simulink model "demo_zynq"  (R2019b)
settings: Solver=FixedStepAuto  StartTime=0.0  StopTime=0.02  RelTol=1e-3  EnableMultiTasking=on
InitFcn:
  | Ts_FPGA = 1/25e6;   % FPGA sampling time (clock)
  | Ts_ADC_comm = 1/2.5e6;   % ADC communication period
  | Ts_ADC_sample = 70e-6;   % ADC sampling time
  | 
  | Ts_ARM = 210e-6;   % ARM execution period
  | 
  | DeadTime = 1e-6;   % deadtime for output signals
  | 
  | FIFO_length = 1000;   % number of fifo samples
  | 
  | Ts_SRO = 1/8e6; % communication time for the shift register outputs
model workspace (MAT data in the model file):
  mwTaskManagerKernelLatency = 1e-06
undefined symbols (not defined in the file): pos_bit
libraries: simulink x43, hdlsllib x24
(part 1 of 2)
settings Model: Creator=drift  LastModifiedBy=lcase
settings SolverCC: PositivePriorityOrder=on
settings OptimizationCC: BlockReduction=off  ConditionallyExecuteInputs=off  DefaultParameterBehavior=Inlined  PassReuseOutputArgsAs=Individual arguments  ZeroExternalMemoryAtStartup=off  ZeroInternalMemoryAtStartup=off  MaxStackSize=64  OptimizationLevel=level1  OptimizationCustomize=off  EfficientTunableParamExpr=on
settings DebuggingCC: AlgebraicLoopMsg=error  ParameterTunabilityLossMsg=error
settings HardwareCC: ProdBitPerPointer=32  ProdBitPerSizeT=32  ProdBitPerPtrDiffT=32  ProdLargestAtomicFloat=None  ProdIntDivRoundTo=Undefined  ProdEndianess=Unspecified  ProdWordSize=32  ProdHWDeviceType=ASIC/FPGA->ASIC/FPGA  TargetBitPerPointer=64  TargetBitPerSizeT=64  TargetBitPerPtrDiffT=64  TargetLongLongMode=on  TargetIntDivRoundTo=Zero  TargetEndianess=LittleEndian  TargetWordSize=64  TargetHWDeviceType=Custom Processor->MATLAB Host Computer  ProdEqTarget=off  HardwareBoardFeatureSet=SoCBlockset
settings SFSimCC: MATLABDynamicMemAlloc=off
settings RTWCC: SystemTargetFile=ert.tlc  HardwareBoard=Custom Hardware Board  TLCOptions="-aInlineSetEventsForThisBaseRateFcn=TLC_FALSE -aSuppressMultiTaskScheduler=TLC_FALSE  -aRateBasedStepFcn=0"  TemplateMakefile=ert_default_tmf
settings CodeAppCC: ForceParamTrailComments=on  IgnoreCustomStorageClasses=off  OperatorAnnotations=on  SimulinkDataObjDesc=on  SFDataObjDesc=on  InsertBlockDesc=on

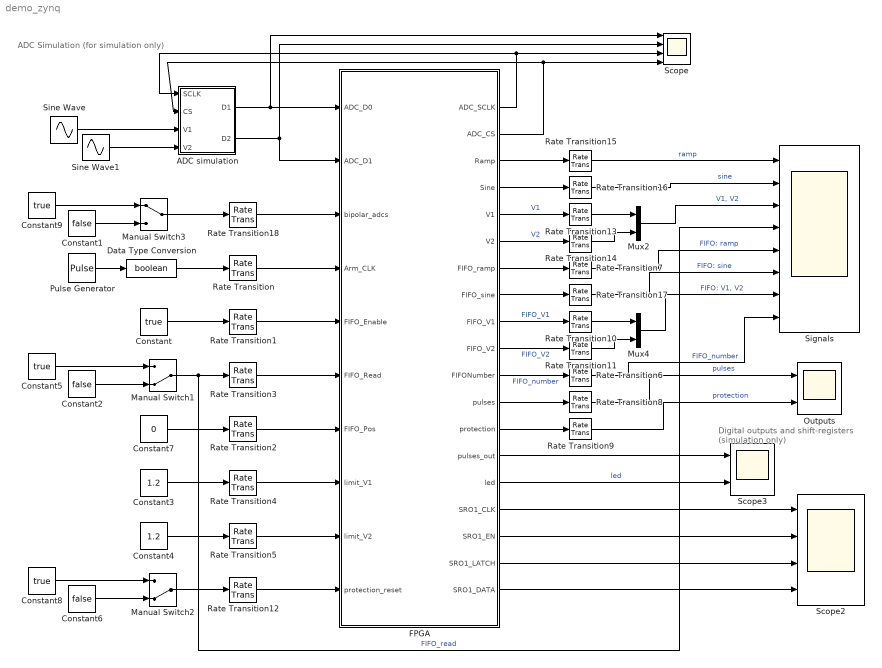
== system demo_zynq ==
  note: Digital outputs
      |                        and shift-registers
      |                          (simulation only)
  note: ADC Simulation
      | (for simulation only)
  ADC simulation : Subsystem
  Constant{,5,8..9} (4 alike) : Constant  Value=true  SampleTime=Ts_ARM
  Constant1 : Constant  Value=false  SampleTime=Ts_ARM
  Constant2 : Constant  Value=false  SampleTime=Ts_ARM
  Constant3 : Constant  Value=1.2  OutDataTypeStr=Inherit: Inherit via back propagation  SampleTime=Ts_ARM
  Constant4 : Constant  Value=1.2  OutDataTypeStr=Inherit: Inherit via back propagation  SampleTime=Ts_ARM
  Constant6 : Constant  Value=false  SampleTime=Ts_ARM
  Constant7 : Constant  Value=0  OutDataTypeStr=Inherit: Inherit via back propagation  SampleTime=Ts_ARM
  Data Type Conversion : DataTypeConversion  OutDataTypeStr=boolean
  FPGA : Subsystem  TreatAsAtomicUnit=on
  Manual Switch1 : ManualSwitch  CurrentSetting=0
  Manual Switch2 : ManualSwitch  CurrentSetting=0
  Manual Switch3 : ManualSwitch
  Mux2 : Mux  Inputs=2
  Mux4 : Mux  Inputs=2
  Outputs : Scope  NumInputPorts=2
  Pulse Generator : DiscretePulseGenerator  SampleTime=Ts_ARM
  Rate Transition{,1..5,12,18} (8 alike) : RateTransition  Integrity=off
  Rate Transition{6..11,13..17} (11 alike) : RateTransition  Integrity=off  OutPortSampleTime=Ts_ARM
  Scope : Scope  NumInputPorts=4
  Scope2 : Scope  NumInputPorts=4
  Scope3 : Scope  NumInputPorts=2
  Signals : Scope  NumInputPorts=8
  Sine Wave : Sin  Bias=1.65  Frequency=2*pi*50  SampleTime=Ts_FPGA
  Sine Wave1 : Sin  Bias=1.65  Frequency=2*pi*50  Phase=-pi/2  SampleTime=Ts_FPGA
  wires:
  Pulse Generator/1 -> Data Type Conversion/1
  Rate Transition/1 -> FPGA/4(Arm_CLK)
  Data Type Conversion/1 -> Rate Transition/1
  Constant/1 -> Rate Transition1/1
  Rate Transition1/1 -> FPGA/5(FIFO_Enable)
  Manual Switch1/1 -> Signals/4, Rate Transition3/1  "FIFO_read"
  Rate Transition3/1 -> FPGA/6(FIFO_Read)
  Constant2/1 -> Manual Switch1/2
  Rate Transition4/1 -> FPGA/8(limit_V1)
  Constant3/1 -> Rate Transition4/1
  Constant4/1 -> Rate Transition5/1
  Rate Transition5/1 -> FPGA/9(limit_V2)
  Constant6/1 -> Manual Switch2/2
  Constant8/1 -> Manual Switch2/1
  Rate Transition12/1 -> FPGA/10(protection_reset)
  Manual Switch2/1 -> Rate Transition12/1
  FPGA/1(ADC_SCLK) -> Scope/3, ADC simulation/1(SCLK)
  FPGA/2(ADC_CS) -> ADC simulation/2(CS), Scope/4
  ADC simulation/1(D1) -> Scope/1, FPGA/1(ADC_D0)
  ADC simulation/2(D2) -> FPGA/2(ADC_D1), Scope/2
  FPGA/5(V1) -> Rate Transition13/1  "V1"
  FPGA/6(V2) -> Rate Transition14/1  "V2"
  FPGA/13(protection) -> Rate Transition9/1
  FPGA/11(FIFONumber) -> Rate Transition6/1  "FIFO_number"
  FPGA/9(FIFO_V1) -> Rate Transition10/1  "FIFO_V1"
  FPGA/10(FIFO_V2) -> Rate Transition11/1  "FIFO_V2"
  Constant7/1 -> Rate Transition2/1
  Rate Transition2/1 -> FPGA/7(FIFO_Pos)
  Constant5/1 -> Manual Switch1/1
  FPGA/12(pulses) -> Rate Transition8/1
  FPGA/16(SRO1_CLK) -> Scope2/1
  FPGA/17(SRO1_EN) -> Scope2/2
  FPGA/18(SRO1_LATCH) -> Scope2/3
  FPGA/19(SRO1_DATA) -> Scope2/4
  FPGA/14(pulses_out) -> Scope3/1
  FPGA/15(led) -> Scope3/2  "led"
  FPGA/3(Ramp) -> Rate Transition15/1
  FPGA/7(FIFO_ramp) -> Rate Transition7/1
  FPGA/4(Sine) -> Rate Transition16/1
  FPGA/8(FIFO_sine) -> Rate Transition17/1
  Rate Transition18/1 -> FPGA/3(bipolar_adcs)
  Manual Switch3/1 -> Rate Transition18/1
  Rate Transition16/1 -> Signals/2  "sine"
  Rate Transition15/1 -> Signals/1  "ramp"
  Rate Transition13/1 -> Mux2/1
  Rate Transition14/1 -> Mux2/2
  Mux2/1 -> Signals/3  "V1, V2"
  Rate Transition11/1 -> Mux4/2
  Rate Transition10/1 -> Mux4/1
  Rate Transition7/1 -> Signals/5  "FIFO: ramp"
  Rate Transition17/1 -> Signals/6  "FIFO: sine"
  Mux4/1 -> Signals/7  "FIFO: V1, V2"
  Rate Transition8/1 -> Outputs/1  "pulses"
  Rate Transition9/1 -> Outputs/2  "protection"
  Rate Transition6/1 -> Signals/8  "FIFO_number"
  Constant9/1 -> Manual Switch3/1
  Constant1/1 -> Manual Switch3/2
  Sine Wave1/1 -> ADC simulation/4(V2)
  Sine Wave/1 -> ADC simulation/3(V1)

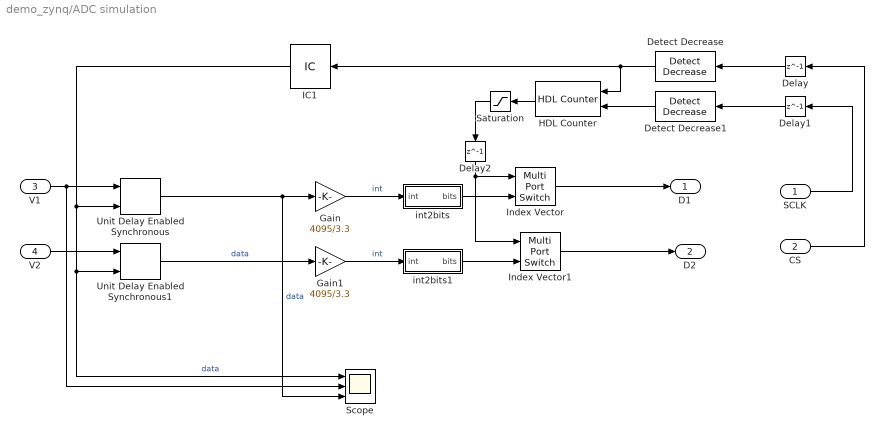
== system demo_zynq/ADC simulation ==
  SCLK : Inport
  CS : Inport  Port=2
  V1 : Inport  Port=3
  V2 : Inport  Port=4
  Delay : Delay  DelayLength=1
  Delay1 : Delay  DelayLength=1
  Delay2 : Delay  DelayLength=1
  Detect Decrease : simulink/Logic and Bit Operations/Detect Decrease  vinit=0.0  OutDataTypeStr=boolean
  Detect Decrease1 : simulink/Logic and Bit Operations/Detect Decrease  vinit=0.0  OutDataTypeStr=boolean
  Gain : Gain  Gain=4095/3.3  OutDataTypeStr=fixdt(0,12,0)  RndMeth=Nearest  SaturateOnIntegerOverflow=on
  Gain1 : Gain  Gain=4095/3.3  OutDataTypeStr=fixdt(0,12,0)  RndMeth=Nearest  SaturateOnIntegerOverflow=on
  HDL Counter : hdlsllib/Sources/HDL Counter  CountType=Free running  CountInit=0  CountStep=1  CountMax=25  CountFromType=Initial value  CountFrom=0  CountResetPort=on  CountLoadPort=off  CountEnbPort=on  CountDirPort=off  CountDataType=Unsigned  CountWordLen=8  CountFracLen=0  CountSampTime=Ts_FPGA
      settings: SourceProductName=Simulink
  IC1 : InitialCondition  Value=true
  Index Vector : MultiPortSwitch  DataPortOrder=Zero-based contiguous  Inputs=1  zeroidx=on
  Index Vector1 : MultiPortSwitch  DataPortOrder=Zero-based contiguous  Inputs=1  zeroidx=on
  Saturation : Saturate  UpperLimit=16  LowerLimit=0
  Scope : Scope  NumInputPorts=3
  Unit Delay Enabled Synchronous : hdlsllib/Discrete/Unit Delay Enabled Synchronous  InitialCondition=0.0  SampleTime=-1
      settings: SourceProductName=Simulink  SourceProductBaseCode=SL
  Unit Delay Enabled Synchronous1 : hdlsllib/Discrete/Unit Delay Enabled Synchronous  InitialCondition=0.0  SampleTime=-1
      settings: SourceProductName=Simulink  SourceProductBaseCode=SL
  int2bits : Subsystem
  int2bits1 : Subsystem
  D1 : Outport
  D2 : Outport  Port=2
  wires:
  Delay1/1 -> Detect Decrease1/1
  V1/1 -> Unit Delay Enabled Synchronous/1, Scope/2
  HDL Counter/1 -> Saturation/1
  Detect Decrease1/1 -> HDL Counter/2
  Delay/1 -> Detect Decrease/1
  Gain/1 -> int2bits/1(int)  "int"
  Unit Delay Enabled Synchronous/1 -> Scope/3, Gain/1  "data"
  int2bits/1(bits) -> Index Vector/2
  Saturation/1 -> Delay2/1
  Index Vector/1 -> D1/1
  SCLK/1 -> Delay1/1
  CS/1 -> Delay/1
  Gain1/1 -> int2bits1/1(int)  "int"
  V2/1 -> Unit Delay Enabled Synchronous1/1
  Index Vector1/1 -> D2/1
  int2bits1/1(bits) -> Index Vector1/2
  Delay2/1 -> Index Vector1/1, Index Vector/1
  Detect Decrease/1 -> IC1/1, HDL Counter/1
  Unit Delay Enabled Synchronous1/1 -> Gain1/1  "data"
  IC1/1 -> Unit Delay Enabled Synchronous/2, Unit Delay Enabled Synchronous1/2, Scope/1  "data"

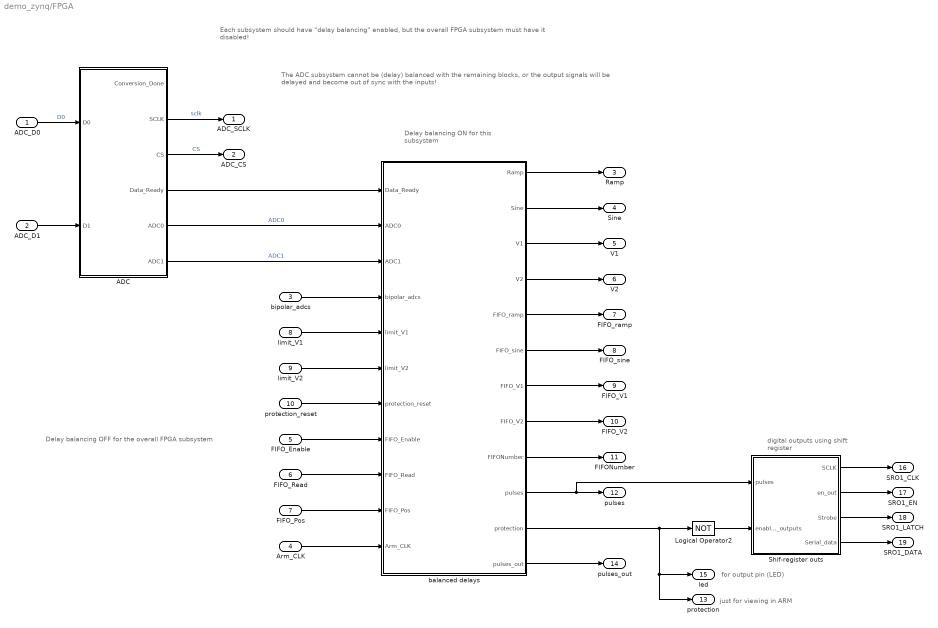
== system demo_zynq/FPGA ==
  note: The ADC subsystem cannot be (delay) balanced with the remaining blocks,
      | or the output signals will be delayed and become out of sync with the inputs!
  note: Each subsystem should have "delay balancing" enabled,
      | but the overall FPGA subsystem must have it disabled!
  note: Delay balancing ON
      | for this subsystem
  note: Delay balancing OFF
      | for the overall FPGA subsystem
  note: digital outputs
      | using shift register
  note: just for viewing in ARM
  note: for output pin (LED)
  ADC_D0 : Inport  OutDataTypeStr=boolean  PortDimensions=1
  ADC_D1 : Inport  Port=2  OutDataTypeStr=boolean  PortDimensions=1
  bipolar_adcs : Inport  Port=3  OutDataTypeStr=boolean  PortDimensions=1
  Arm_CLK : Inport  Port=4  OutDataTypeStr=boolean  PortDimensions=1
  FIFO_Enable : Inport  Port=5  OutDataTypeStr=boolean
  FIFO_Read : Inport  Port=6  OutDataTypeStr=boolean
  FIFO_Pos : Inport  Port=7  OutDataTypeStr=uint32
  limit_V1 : Inport  Port=8  OutDataTypeStr=fixdt(1,32,29)
  limit_V2 : Inport  Port=9  OutDataTypeStr=fixdt(1,32,29)
  protection_reset : Inport  Port=10  OutDataTypeStr=boolean
  ADC : Subsystem
  Logical Operator2 : Logic  Operator=NOT  AllPortsSameDT=off  OutDataTypeStr=boolean
  Shif-register outs : Subsystem  TreatAsAtomicUnit=on  mask{Nbits_SRO=8}
      mask prompts: Nbits_SRO "Number of bits to send"
  balanced delays : Subsystem
  ADC_SCLK : Outport  VectorParamsAs1DForOutWhenUnconnected=off
  ADC_CS : Outport  Port=2  VectorParamsAs1DForOutWhenUnconnected=off
  Ramp : Outport  Port=3  VectorParamsAs1DForOutWhenUnconnected=off
  Sine : Outport  Port=4  VectorParamsAs1DForOutWhenUnconnected=off
  V1 : Outport  Port=5  VectorParamsAs1DForOutWhenUnconnected=off
  V2 : Outport  Port=6  VectorParamsAs1DForOutWhenUnconnected=off
  FIFO_ramp : Outport  Port=7  VectorParamsAs1DForOutWhenUnconnected=off
  FIFO_sine : Outport  Port=8  VectorParamsAs1DForOutWhenUnconnected=off
  FIFO_V1 : Outport  Port=9  VectorParamsAs1DForOutWhenUnconnected=off
  FIFO_V2 : Outport  Port=10  VectorParamsAs1DForOutWhenUnconnected=off
  FIFONumber : Outport  Port=11  VectorParamsAs1DForOutWhenUnconnected=off
  pulses : Outport  Port=12  VectorParamsAs1DForOutWhenUnconnected=off
  protection : Outport  Port=13  VectorParamsAs1DForOutWhenUnconnected=off
  pulses_out : Outport  Port=14  VectorParamsAs1DForOutWhenUnconnected=off
  led : Outport  Port=15  VectorParamsAs1DForOutWhenUnconnected=off
  SRO1_CLK : Outport  Port=16
  SRO1_EN : Outport  Port=17
  SRO1_LATCH : Outport  Port=18
  SRO1_DATA : Outport  Port=19
  wires:
  ADC_D0/1 -> ADC/1(D0)  "D0"
  ADC_D1/1 -> ADC/2(D1)
  ADC/3(CS) -> ADC_CS/1  "CS"
  ADC/2(SCLK) -> ADC_SCLK/1  "sclk"
  ADC/4(Data_Ready) -> balanced delays/1(Data_Ready)
  ADC/5(ADC0) -> balanced delays/2(ADC0)  "ADC0"
  ADC/6(ADC1) -> balanced delays/3(ADC1)  "ADC1"
  bipolar_adcs/1 -> balanced delays/4(bipolar_adcs)
  limit_V1/1 -> balanced delays/5(limit_V1)
  limit_V2/1 -> balanced delays/6(limit_V2)
  protection_reset/1 -> balanced delays/7(protection_reset)
  FIFO_Enable/1 -> balanced delays/8(FIFO_Enable)
  FIFO_Read/1 -> balanced delays/9(FIFO_Read)
  FIFO_Pos/1 -> balanced delays/10(FIFO_Pos)
  Arm_CLK/1 -> balanced delays/11(Arm_CLK)
  balanced delays/1(Ramp) -> Ramp/1
  balanced delays/2(Sine) -> Sine/1
  balanced delays/3(V1) -> V1/1
  balanced delays/4(V2) -> V2/1
  balanced delays/5(FIFO_ramp) -> FIFO_ramp/1
  balanced delays/6(FIFO_sine) -> FIFO_sine/1
  balanced delays/7(FIFO_V1) -> FIFO_V1/1
  balanced delays/8(FIFO_V2) -> FIFO_V2/1
  balanced delays/9(FIFONumber) -> FIFONumber/1
  balanced delays/12(pulses_out) -> pulses_out/1
  Shif-register outs/1(SCLK) -> SRO1_CLK/1
  Shif-register outs/2(en_out) -> SRO1_EN/1
  Shif-register outs/3("Strobe ") -> SRO1_LATCH/1
  Shif-register outs/4(Serial_data) -> SRO1_DATA/1
  balanced delays/11(protection) -> protection/1, led/1, Logical Operator2/1
  balanced delays/10(pulses) -> pulses/1, Shif-register outs/1(pulses)
  Logical Operator2/1 -> Shif-register outs/2(enable_outputs)

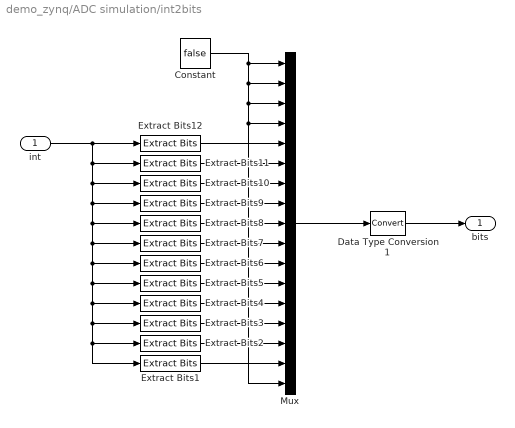
== system demo_zynq/ADC simulation/int2bits ==
  int : Inport
  Constant : Constant  Value=false  OutDataTypeStr=fixdt(0,1,0)
  Data Type Conversion1 : DataTypeConversion
  Extract Bits1 : simulink/Logic and Bit Operations/Extract Bits  bitsToExtract=Range of bits  numBits=8  bitIdxRange=0  outScalingMode=Preserve fixed-point scaling
      settings: SourceProductName=Simulink
  Extract Bits10 : simulink/Logic and Bit Operations/Extract Bits  bitsToExtract=Range of bits  numBits=8  bitIdxRange=9  outScalingMode=Treat bit field as an integer
      settings: SourceProductName=Simulink
  Extract Bits11 : simulink/Logic and Bit Operations/Extract Bits  bitsToExtract=Range of bits  numBits=8  bitIdxRange=10  outScalingMode=Treat bit field as an integer
      settings: SourceProductName=Simulink
  Extract Bits12 : simulink/Logic and Bit Operations/Extract Bits  bitsToExtract=Range of bits  numBits=8  bitIdxRange=11  outScalingMode=Treat bit field as an integer
      settings: SourceProductName=Simulink
  Extract Bits2 : simulink/Logic and Bit Operations/Extract Bits  bitsToExtract=Range of bits  numBits=8  bitIdxRange=1  outScalingMode=Treat bit field as an integer
      settings: SourceProductName=Simulink
  Extract Bits3 : simulink/Logic and Bit Operations/Extract Bits  bitsToExtract=Range of bits  numBits=8  bitIdxRange=2  outScalingMode=Treat bit field as an integer
      settings: SourceProductName=Simulink
  Extract Bits4 : simulink/Logic and Bit Operations/Extract Bits  bitsToExtract=Range of bits  numBits=8  bitIdxRange=3  outScalingMode=Treat bit field as an integer
      settings: SourceProductName=Simulink
  Extract Bits5 : simulink/Logic and Bit Operations/Extract Bits  bitsToExtract=Range of bits  numBits=8  bitIdxRange=4  outScalingMode=Treat bit field as an integer
      settings: SourceProductName=Simulink
  Extract Bits6 : simulink/Logic and Bit Operations/Extract Bits  bitsToExtract=Range of bits  numBits=8  bitIdxRange=5  outScalingMode=Treat bit field as an integer
      settings: SourceProductName=Simulink
  Extract Bits7 : simulink/Logic and Bit Operations/Extract Bits  bitsToExtract=Range of bits  numBits=8  bitIdxRange=6  outScalingMode=Treat bit field as an integer
      settings: SourceProductName=Simulink
  Extract Bits8 : simulink/Logic and Bit Operations/Extract Bits  bitsToExtract=Range of bits  numBits=8  bitIdxRange=7  outScalingMode=Treat bit field as an integer
      settings: SourceProductName=Simulink
  Extract Bits9 : simulink/Logic and Bit Operations/Extract Bits  bitsToExtract=Range of bits  numBits=8  bitIdxRange=8  outScalingMode=Treat bit field as an integer
      settings: SourceProductName=Simulink
  Mux : Mux  Inputs=17
  bits : Outport
  wires:
  Extract Bits12/1 -> Mux/5
  Extract Bits8/1 -> Mux/9
  Extract Bits2/1 -> Mux/15
  Extract Bits5/1 -> Mux/12
  Extract Bits9/1 -> Mux/8
  int/1 -> Extract Bits12/1, Extract Bits11/1, Extract Bits10/1, Extract Bits9/1, Extract Bits8/1, Extract Bits7/1, Extract Bits6/1, Extract Bits5/1, Extract Bits4/1, Extract Bits3/1, Extract Bits2/1, Extract Bits1/1
  Extract Bits11/1 -> Mux/6
  Extract Bits7/1 -> Mux/10
  Extract Bits10/1 -> Mux/7
  Extract Bits4/1 -> Mux/13
  Extract Bits3/1 -> Mux/14
  Extract Bits6/1 -> Mux/11
  Extract Bits1/1 -> Mux/16
  Mux/1 -> Data Type Conversion1/1
  Constant/1 -> Mux/1, Mux/2, Mux/3, Mux/17, Mux/4
  Data Type Conversion1/1 -> bits/1

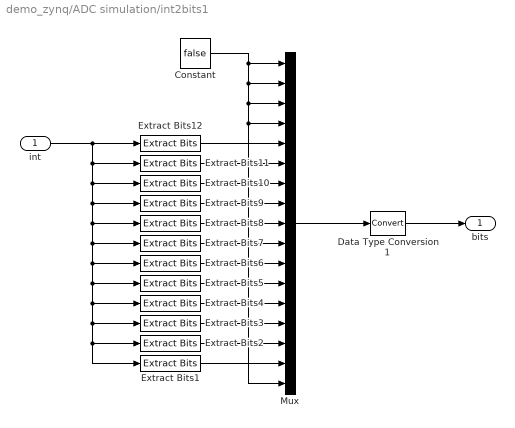
== system demo_zynq/ADC simulation/int2bits1 ==
  int : Inport
  Constant : Constant  Value=false  OutDataTypeStr=fixdt(0,1,0)
  Data Type Conversion1 : DataTypeConversion
  Extract Bits1 : simulink/Logic and Bit Operations/Extract Bits  bitsToExtract=Range of bits  numBits=8  bitIdxRange=0  outScalingMode=Preserve fixed-point scaling
      settings: SourceProductName=Simulink
  Extract Bits10 : simulink/Logic and Bit Operations/Extract Bits  bitsToExtract=Range of bits  numBits=8  bitIdxRange=9  outScalingMode=Treat bit field as an integer
      settings: SourceProductName=Simulink
  Extract Bits11 : simulink/Logic and Bit Operations/Extract Bits  bitsToExtract=Range of bits  numBits=8  bitIdxRange=10  outScalingMode=Treat bit field as an integer
      settings: SourceProductName=Simulink
  Extract Bits12 : simulink/Logic and Bit Operations/Extract Bits  bitsToExtract=Range of bits  numBits=8  bitIdxRange=11  outScalingMode=Treat bit field as an integer
      settings: SourceProductName=Simulink
  Extract Bits2 : simulink/Logic and Bit Operations/Extract Bits  bitsToExtract=Range of bits  numBits=8  bitIdxRange=1  outScalingMode=Treat bit field as an integer
      settings: SourceProductName=Simulink
  Extract Bits3 : simulink/Logic and Bit Operations/Extract Bits  bitsToExtract=Range of bits  numBits=8  bitIdxRange=2  outScalingMode=Treat bit field as an integer
      settings: SourceProductName=Simulink
  Extract Bits4 : simulink/Logic and Bit Operations/Extract Bits  bitsToExtract=Range of bits  numBits=8  bitIdxRange=3  outScalingMode=Treat bit field as an integer
      settings: SourceProductName=Simulink
  Extract Bits5 : simulink/Logic and Bit Operations/Extract Bits  bitsToExtract=Range of bits  numBits=8  bitIdxRange=4  outScalingMode=Treat bit field as an integer
      settings: SourceProductName=Simulink
  Extract Bits6 : simulink/Logic and Bit Operations/Extract Bits  bitsToExtract=Range of bits  numBits=8  bitIdxRange=5  outScalingMode=Treat bit field as an integer
      settings: SourceProductName=Simulink
  Extract Bits7 : simulink/Logic and Bit Operations/Extract Bits  bitsToExtract=Range of bits  numBits=8  bitIdxRange=6  outScalingMode=Treat bit field as an integer
      settings: SourceProductName=Simulink
  Extract Bits8 : simulink/Logic and Bit Operations/Extract Bits  bitsToExtract=Range of bits  numBits=8  bitIdxRange=7  outScalingMode=Treat bit field as an integer
      settings: SourceProductName=Simulink
  Extract Bits9 : simulink/Logic and Bit Operations/Extract Bits  bitsToExtract=Range of bits  numBits=8  bitIdxRange=8  outScalingMode=Treat bit field as an integer
      settings: SourceProductName=Simulink
  Mux : Mux  Inputs=17
  bits : Outport
  wires:
  Data Type Conversion1/1 -> bits/1
  Constant/1 -> Mux/4, Mux/17, Mux/3, Mux/2, Mux/1
  Mux/1 -> Data Type Conversion1/1
  Extract Bits1/1 -> Mux/16
  Extract Bits6/1 -> Mux/11
  Extract Bits3/1 -> Mux/14
  Extract Bits4/1 -> Mux/13
  Extract Bits10/1 -> Mux/7
  Extract Bits7/1 -> Mux/10
  Extract Bits11/1 -> Mux/6
  int/1 -> Extract Bits1/1, Extract Bits2/1, Extract Bits3/1, Extract Bits4/1, Extract Bits5/1, Extract Bits6/1, Extract Bits7/1, Extract Bits8/1, Extract Bits9/1, Extract Bits10/1, Extract Bits11/1, Extract Bits12/1
  Extract Bits9/1 -> Mux/8
  Extract Bits5/1 -> Mux/12
  Extract Bits2/1 -> Mux/15
  Extract Bits8/1 -> Mux/9
  Extract Bits12/1 -> Mux/5

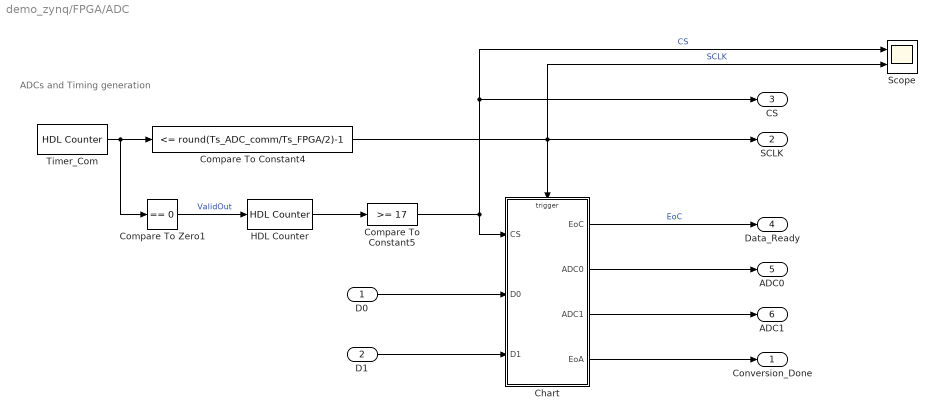
== system demo_zynq/FPGA/ADC ==
  note: ADCs and Timing generation
  D0 : Inport  OutDataTypeStr=boolean  PortDimensions=1
  D1 : Inport  Port=2  OutDataTypeStr=boolean  PortDimensions=1
  Chart : Stateflow chart  TreatAsAtomicUnit=on
  Compare To Constant4 : simulink/Logic and Bit Operations/Compare To Constant  relop=<=  const=round(Ts_ADC_comm/Ts_FPGA/2)-1  OutDataTypeStr=boolean
  Compare To Constant5 : simulink/Logic and Bit Operations/Compare To Constant  relop=>=  const=17  OutDataTypeStr=boolean
  Compare To Zero1 : simulink/Logic and Bit Operations/Compare To Zero  relop===  OutDataTypeStr=boolean
  HDL Counter : hdlsllib/Sources/HDL Counter  CountType=Count limited  CountInit=0  CountStep=1  CountMax=round(Ts_ADC_sample/Ts_ADC_comm)-1  CountFromType=Initial value  CountFrom=0  CountResetPort=off  CountLoadPort=off  CountEnbPort=on  CountDirPort=off  CountDataType=Unsigned  CountWordLen=32  CountFracLen=0  CountSampTime=Ts_FPGA
      settings: SourceProductName=Simulink
  Scope : Scope  NumInputPorts=2
  Timer_Com : hdlsllib/Sources/HDL Counter  CountType=Count limited  CountInit=0  CountStep=1  CountMax=round(Ts_ADC_comm/Ts_FPGA)-1  CountFromType=Initial value  CountFrom=0  CountResetPort=off  CountLoadPort=off  CountEnbPort=off  CountDirPort=off  CountDataType=Unsigned  CountWordLen=32  CountFracLen=0  CountSampTime=Ts_FPGA
  Conversion_Done : Outport
  SCLK : Outport  Port=2  OutDataTypeStr=boolean  PortDimensions=1
  CS : Outport  Port=3  OutDataTypeStr=boolean  PortDimensions=1
  Data_Ready : Outport  Port=4
  ADC0 : Outport  Port=5
  ADC1 : Outport  Port=6
  wires:
  Timer_Com/1 -> Compare To Zero1/1, Compare To Constant4/1
  Compare To Constant5/1 -> Scope/1, CS/1, Chart/1(CS)  "CS"
  Chart/1(EoC) -> Data_Ready/1  "EoC"
  D0/1 -> Chart/2(D0)
  Compare To Constant4/1 -> Scope/2, SCLK/1, Chart/Trigger  "SCLK"
  HDL Counter/1 -> Compare To Constant5/1
  Compare To Zero1/1 -> HDL Counter/1  "ValidOut"
  D1/1 -> Chart/3(D1)
  Chart/4(EoA) -> Conversion_Done/1
  Chart/2(ADC0) -> ADC0/1
  Chart/3(ADC1) -> ADC1/1

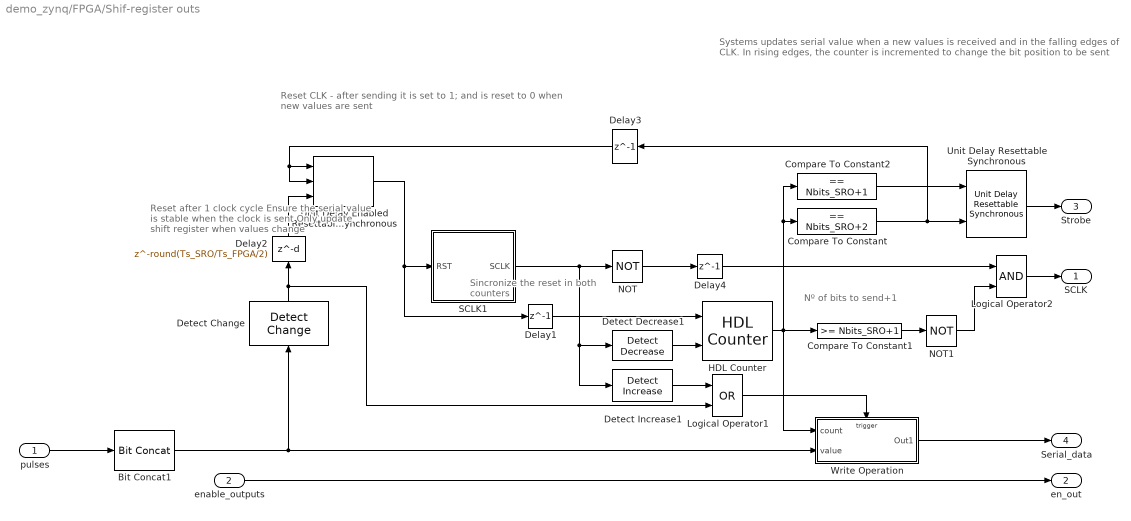
== system demo_zynq/FPGA/Shif-register outs ==
  note: Nº of bits to send+1
  note: Reset after 1
      | clock cycle
      |
      | Ensure the serial
      | value is stable
      | when the clock
      | is sent
      |
      | Only update shift
      | register when
      | values change
  note: Reset CLK - after sending it is set to 1;
      | and is reset to 0 when new values are sent
  note: Systems updates serial value when a new values is received and in
      | the falling edges of CLK.
      | In rising edges, the counter is incremented to change the
      | bit position to be sent
  note: Sincronize the reset
      | in both counters
  pulses : Inport
  enable_outputs : Inport  Port=2
  Bit Concat1 : hdlsllib/Logic and Bit Operations/Bit Concat  numInputs=1
  Compare To Constant : simulink/Logic and Bit Operations/Compare To Constant  relop===  const=Nbits_SRO+2  OutDataTypeStr=boolean
  Compare To Constant1 : simulink/Logic and Bit Operations/Compare To Constant  relop=>=  const=Nbits_SRO+1  OutDataTypeStr=boolean
  Compare To Constant2 : simulink/Logic and Bit Operations/Compare To Constant  relop===  const=Nbits_SRO+1  OutDataTypeStr=boolean
  Delay1 : Delay  DelayLength=1
  Delay2 : Delay  DelayLength=round(Ts_SRO/Ts_FPGA/2)
  Delay3 : Delay  DelayLength=1  InitialCondition=1
  Delay4 : Delay  DelayLength=1
  Detect Change : simulink/Logic and Bit Operations/Detect Change  vinit=0  OutDataTypeStr=boolean
  Detect Decrease1 : simulink/Logic and Bit Operations/Detect Decrease  vinit=0.0  OutDataTypeStr=boolean
  Detect Increase1 : simulink/Logic and Bit Operations/Detect Increase  vinit=0.0  OutDataTypeStr=boolean
  HDL Counter : hdlsllib/Sources/HDL Counter  CountType=Free running  CountInit=0  CountStep=1  CountMax=16  CountFromType=Initial value  CountFrom=0  CountResetPort=on  CountLoadPort=off  CountEnbPort=on  CountDirPort=off  CountDataType=Unsigned  CountWordLen=8  CountFracLen=0  CountSampTime=1
  Logical Operator1 : Logic  Operator=OR  AllPortsSameDT=off  OutDataTypeStr=boolean
  Logical Operator2 : Logic  AllPortsSameDT=off  OutDataTypeStr=boolean
  NOT : Logic  Operator=NOT  IconShape=distinctive  AllPortsSameDT=off  OutDataTypeStr=boolean
  NOT1 : Logic  Operator=NOT  IconShape=distinctive  AllPortsSameDT=off  OutDataTypeStr=boolean
  SCLK1 : Subsystem
  Unit Delay Enabled Resettable Synchronous : hdlsllib/Discrete/Unit Delay Enabled Resettable Synchronous  InitialCondition=0.0  SampleTime=-1
      settings: SourceProductBaseCode=SL
  Unit Delay Resettable Synchronous : hdlsllib/Discrete/Unit Delay Resettable Synchronous  InitialCondition=0.0  SampleTime=-1
      settings: SourceProductBaseCode=SL
  Write Operation : Subsystem  TreatAsAtomicUnit=on
  SCLK : Outport
  en_out : Outport  Port=2
  "Strobe " : Outport  Port=3
  Serial_data : Outport  Port=4
  wires:
  NOT/1 -> Delay4/1
  Compare To Constant1/1 -> NOT1/1
  Logical Operator2/1 -> SCLK/1
  SCLK1/1(SCLK) -> Detect Decrease1/1, Detect Increase1/1, NOT/1
  Delay3/1 -> Unit Delay Enabled Resettable Synchronous/2, Unit Delay Enabled Resettable Synchronous/1
  Unit Delay Resettable Synchronous/1 -> "Strobe "/1
  HDL Counter/1 -> Compare To Constant1/1, Write Operation/1(count), Compare To Constant2/1, Compare To Constant/1
  enable_outputs/1 -> en_out/1
  Detect Change/1 -> Delay2/1, Logical Operator1/2
  Write Operation/1(Out1) -> Serial_data/1
  NOT1/1 -> Logical Operator2/2
  Detect Increase1/1 -> Logical Operator1/1
  Logical Operator1/1 -> Write Operation/Trigger
  Unit Delay Enabled Resettable Synchronous/1 -> Delay1/1, SCLK1/1(RST)
  Delay2/1 -> Unit Delay Enabled Resettable Synchronous/3
  pulses/1 -> Bit Concat1/1
  Detect Decrease1/1 -> HDL Counter/2
  Delay4/1 -> Logical Operator2/1
  Compare To Constant/1 -> Delay3/1, Unit Delay Resettable Synchronous/2
  Compare To Constant2/1 -> Unit Delay Resettable Synchronous/1
  Delay1/1 -> HDL Counter/1
  Bit Concat1/1 -> Detect Change/1, Write Operation/2(value)

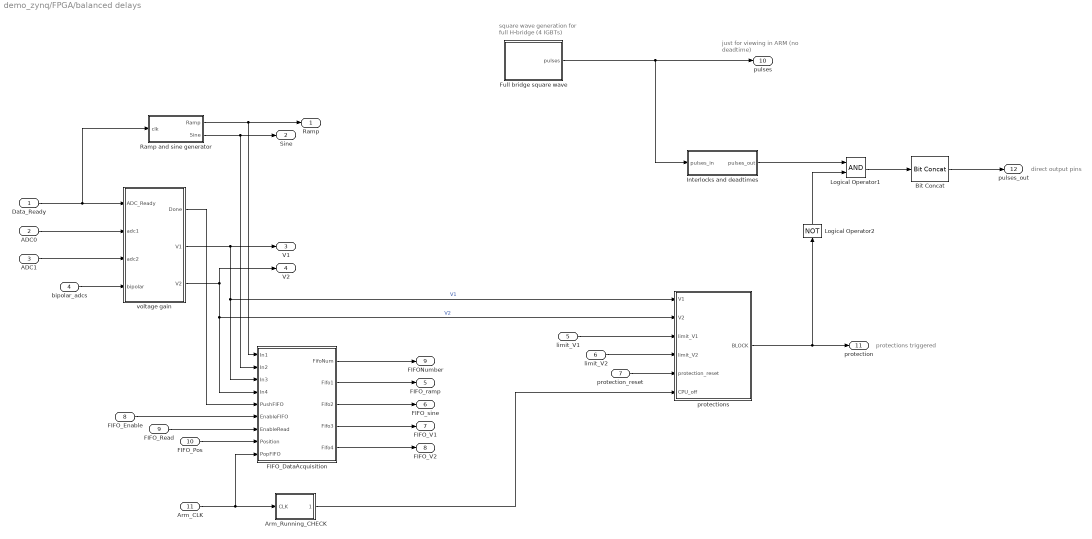
== system demo_zynq/FPGA/balanced delays ==
  note: just for viewing in ARM
      | (no deadtime)
  note: direct output pins
  note: square wave generation
      | for full H-bridge (4 IGBTs)
  note: protections triggered
  Data_Ready : Inport
  ADC0 : Inport  Port=2
  ADC1 : Inport  Port=3
  bipolar_adcs : Inport  Port=4  OutDataTypeStr=boolean  PortDimensions=1
  limit_V1 : Inport  Port=5  OutDataTypeStr=fixdt(1,32,29)
  limit_V2 : Inport  Port=6  OutDataTypeStr=fixdt(1,32,29)
  protection_reset : Inport  Port=7  OutDataTypeStr=boolean
  FIFO_Enable : Inport  Port=8  OutDataTypeStr=boolean
  FIFO_Read : Inport  Port=9  OutDataTypeStr=boolean
  FIFO_Pos : Inport  Port=10  OutDataTypeStr=uint32
  Arm_CLK : Inport  Port=11  OutDataTypeStr=boolean  PortDimensions=1
  Arm_Running_CHECK : Subsystem
  Bit Concat : hdlsllib/Logic and Bit Operations/Bit Concat  numInputs=1
  FIFO_DataAcquisition : Subsystem  SystemSampleTime=70e-6
  Full bridge square wave : Subsystem
  Interlocks and deadtimes : Subsystem
  Logical Operator1 : Logic  AllPortsSameDT=off  OutDataTypeStr=boolean
  Logical Operator2 : Logic  Operator=NOT  AllPortsSameDT=off  OutDataTypeStr=boolean
  Ramp and sine generator : Subsystem
  protections : Subsystem
  voltage gain : Subsystem
  Ramp : Outport  VectorParamsAs1DForOutWhenUnconnected=off
  Sine : Outport  Port=2  VectorParamsAs1DForOutWhenUnconnected=off
  V1 : Outport  Port=3  VectorParamsAs1DForOutWhenUnconnected=off
  V2 : Outport  Port=4  VectorParamsAs1DForOutWhenUnconnected=off
  FIFO_ramp : Outport  Port=5  VectorParamsAs1DForOutWhenUnconnected=off
  FIFO_sine : Outport  Port=6  VectorParamsAs1DForOutWhenUnconnected=off
  FIFO_V1 : Outport  Port=7  VectorParamsAs1DForOutWhenUnconnected=off
  FIFO_V2 : Outport  Port=8  VectorParamsAs1DForOutWhenUnconnected=off
  FIFONumber : Outport  Port=9  VectorParamsAs1DForOutWhenUnconnected=off
  pulses : Outport  Port=10  VectorParamsAs1DForOutWhenUnconnected=off
  protection : Outport  Port=11  VectorParamsAs1DForOutWhenUnconnected=off
  pulses_out : Outport  Port=12  VectorParamsAs1DForOutWhenUnconnected=off
  wires:
  voltage gain/2(V1) -> FIFO_DataAcquisition/3(In3), protections/1(V1), V1/1  "V1"
  FIFO_DataAcquisition/2(Fifo1) -> FIFO_ramp/1
  voltage gain/3("  V2") -> FIFO_DataAcquisition/4(In4), protections/2(V2), V2/1  "V2"
  Data_Ready/1 -> Ramp and sine generator/1(clk), voltage gain/1(ADC_Ready)
  Arm_Running_CHECK/1(ARM_off) -> protections/6(CPU_off)
  voltage gain/1("  Done") -> FIFO_DataAcquisition/5(PushFIFO)
  FIFO_DataAcquisition/1(FifoNum) -> FIFONumber/1
  limit_V2/1 -> protections/4(limit_V2)
  FIFO_DataAcquisition/5(Fifo4) -> FIFO_V2/1
  FIFO_DataAcquisition/3(Fifo2) -> FIFO_sine/1
  protections/1(BLOCK) -> protection/1, Logical Operator2/1
  Full bridge square wave/1(pulses) -> pulses/1, Interlocks and deadtimes/1(pulses_in)
  bipolar_adcs/1 -> voltage gain/4(bipolar)
  ADC0/1 -> voltage gain/2(adc1)
  FIFO_Read/1 -> FIFO_DataAcquisition/7(EnableRead)
  limit_V1/1 -> protections/3(limit_V1)
  Bit Concat/1 -> pulses_out/1
  FIFO_DataAcquisition/4(Fifo3) -> FIFO_V1/1
  Ramp and sine generator/1(Ramp) -> Ramp/1, FIFO_DataAcquisition/1(In1)
  Arm_CLK/1 -> Arm_Running_CHECK/1(CLK), FIFO_DataAcquisition/9(PopFIFO)
  FIFO_Enable/1 -> FIFO_DataAcquisition/6(EnableFIFO)
  protection_reset/1 -> protections/5(protection_reset)
  Interlocks and deadtimes/1(pulses_out) -> Logical Operator1/1
  Ramp and sine generator/2(Sine) -> Sine/1, FIFO_DataAcquisition/2(In2)
  Logical Operator1/1 -> Bit Concat/1
  FIFO_Pos/1 -> FIFO_DataAcquisition/8(Position)
  ADC1/1 -> voltage gain/3(adc2)
  Logical Operator2/1 -> Logical Operator1/2

== system demo_zynq/FPGA/Shif-register outs/SCLK1 ==
  RST : Inport
  Compare To Constant4 : simulink/Logic and Bit Operations/Compare To Constant  relop=<  const=round(Ts_SRO/Ts_FPGA/2)-1  OutDataTypeStr=boolean
  Timer_Com : hdlsllib/Sources/HDL Counter  CountType=Count limited  CountInit=0  CountStep=1  CountMax=round(Ts_SRO/Ts_FPGA)-1  CountFromType=Initial value  CountFrom=0  CountResetPort=on  CountLoadPort=off  CountEnbPort=off  CountDirPort=off  CountDataType=Unsigned  CountWordLen=32  CountFracLen=0  CountSampTime=Ts_FPGA
  SCLK : Outport
  wires:
  Timer_Com/1 -> Compare To Constant4/1
  Compare To Constant4/1 -> SCLK/1  "SCLK"
  RST/1 -> Timer_Com/1

== system demo_zynq/FPGA/Shif-register outs/Write Operation ==
  count : Inport
  value : Inport  Port=2
  Trigger : TriggerPort  VariantControl=Variant  PortDimensions=1
  Bit Shift : hdlsllib/Logic and Bit Operations/Bit Shift  mode=Shift Left Logical  N=1
  Data Type Conversion : DataTypeConversion  OutDataTypeStr=boolean
  Delay : Delay  DelayLength=1  InitialCondition=0
  Extract Bits : simulink/Logic and Bit Operations/Extract Bits  bitsToExtract=Range starting with most significant bit  numBits=1  bitIdxRange=[pos_bit]  outScalingMode=Preserve fixed-point scaling
  Switch : Switch  Threshold=1
  Out1 : Outport  InitialOutput=[0]
  wires:
  Data Type Conversion/1 -> Out1/1
  Delay/1 -> Bit Shift/1
  Extract Bits/1 -> Data Type Conversion/1
  Switch/1 -> Delay/1, Extract Bits/1
  count/1 -> Switch/2
  Bit Shift/1 -> Switch/1
  value/1 -> Switch/3

== system demo_zynq/FPGA/balanced delays/Arm_Running_CHECK ==
  CLK : Inport
  Compare To Constant : simulink/Logic and Bit Operations/Compare To Constant  relop=>  const=round(10*Ts_ARM/Ts_FPGA)  OutDataTypeStr=boolean
  Detect Change : simulink/Logic and Bit Operations/Detect Change  vinit=0  OutDataTypeStr=boolean
  HDL Counter : hdlsllib/Sources/HDL Counter  CountType=Free running  CountInit=0  CountStep=1  CountMax=25  CountFromType=Initial value  CountFrom=0  CountResetPort=on  CountLoadPort=off  CountEnbPort=on  CountDirPort=off  CountDataType=Unsigned  CountWordLen=32  CountFracLen=0  CountSampTime=Ts_FPGA
      settings: SourceProductName=Simulink
  Logical Operator : Logic  Operator=NOT  AllPortsSameDT=off  OutDataTypeStr=boolean
  Scope : Scope  NumInputPorts=3
  ARM_off : Outport
  wires:
  Detect Change/1 -> HDL Counter/1
  Compare To Constant/1 -> Scope/3, Logical Operator/1, ARM_off/1
  HDL Counter/1 -> Scope/2, Compare To Constant/1
  Logical Operator/1 -> HDL Counter/2
  CLK/1 -> Scope/1, Detect Change/1

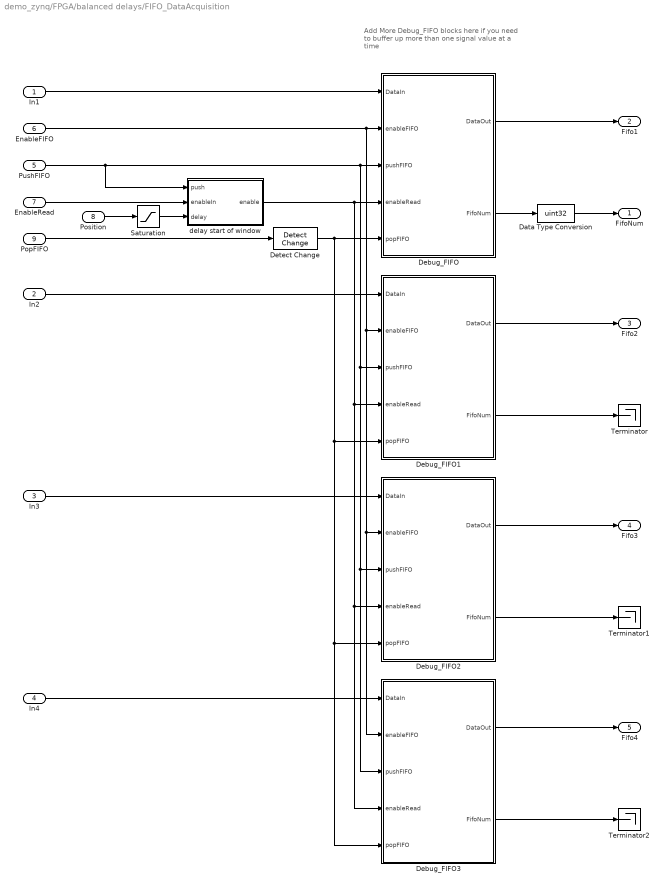
== system demo_zynq/FPGA/balanced delays/FIFO_DataAcquisition ==
  note: Add More Debug_FIFO blocks here if
      | you need to buffer up more than one signal
      | value at a time
  In1 : Inport
  In2 : Inport  Port=2
  In3 : Inport  Port=3
  In4 : Inport  Port=4
  PushFIFO : Inport  Port=5
  EnableFIFO : Inport  Port=6
  EnableRead : Inport  Port=7
  Position : Inport  Port=8
  PopFIFO : Inport  Port=9
  Data Type Conversion : DataTypeConversion  OutDataTypeStr=uint32
  Debug_FIFO : Subsystem
  Debug_FIFO1 : Subsystem
  Debug_FIFO2 : Subsystem
  Debug_FIFO3 : Subsystem
  Detect Change : simulink/Logic and Bit Operations/Detect Change  vinit=0  OutDataTypeStr=boolean
  Saturation : Saturate  UpperLimit=FIFO_length-1  LowerLimit=0
  Terminator : Terminator
  Terminator1 : Terminator
  Terminator2 : Terminator
  delay start of window : Subsystem
  FifoNum : Outport  VectorParamsAs1DForOutWhenUnconnected=off
  Fifo1 : Outport  Port=2  VectorParamsAs1DForOutWhenUnconnected=off
  Fifo2 : Outport  Port=3  VectorParamsAs1DForOutWhenUnconnected=off
  Fifo3 : Outport  Port=4  VectorParamsAs1DForOutWhenUnconnected=off
  Fifo4 : Outport  Port=5  VectorParamsAs1DForOutWhenUnconnected=off
  wires:
  In1/1 -> Debug_FIFO/1(DataIn)
  Debug_FIFO/2(FifoNum) -> Data Type Conversion/1
  Debug_FIFO/1(DataOut) -> Fifo1/1
  PopFIFO/1 -> Detect Change/1
  Debug_FIFO1/1(DataOut) -> Fifo2/1
  Debug_FIFO1/2(FifoNum) -> Terminator/1
  In2/1 -> Debug_FIFO1/1(DataIn)
  EnableRead/1 -> delay start of window/2(enableIn)
  Position/1 -> Saturation/1
  Data Type Conversion/1 -> FifoNum/1
  In3/1 -> Debug_FIFO2/1(DataIn)
  Debug_FIFO2/2(FifoNum) -> Terminator1/1
  Debug_FIFO2/1(DataOut) -> Fifo3/1
  Debug_FIFO3/1(DataOut) -> Fifo4/1
  Debug_FIFO3/2(FifoNum) -> Terminator2/1
  In4/1 -> Debug_FIFO3/1(DataIn)
  Detect Change/1 -> Debug_FIFO3/5(popFIFO), Debug_FIFO2/5(popFIFO), Debug_FIFO1/5(popFIFO), Debug_FIFO/5(popFIFO)
  delay start of window/1(enable) -> Debug_FIFO3/4(enableRead), Debug_FIFO2/4(enableRead), Debug_FIFO1/4(enableRead), Debug_FIFO/4(enableRead)
  EnableFIFO/1 -> Debug_FIFO3/2(enableFIFO), Debug_FIFO2/2(enableFIFO), Debug_FIFO1/2(enableFIFO), Debug_FIFO/2(enableFIFO)
  PushFIFO/1 -> delay start of window/1(push), Debug_FIFO3/3(pushFIFO), Debug_FIFO2/3(pushFIFO), Debug_FIFO1/3(pushFIFO), Debug_FIFO/3(pushFIFO)
  Saturation/1 -> delay start of window/3(delay)

== system demo_zynq/FPGA/balanced delays/Full bridge square wave ==
  Compare To Constant4 : simulink/Logic and Bit Operations/Compare To Constant  relop=<  const=round(0.02/Ts_FPGA/2)-1  OutDataTypeStr=boolean
  Logical Operator : Logic  Operator=NOT  IconShape=distinctive  AllPortsSameDT=off  OutDataTypeStr=boolean
  Mux : Mux
  PWM_counter : hdlsllib/Sources/HDL Counter  CountType=Count limited  CountInit=0  CountStep=1  CountMax=round(0.02/Ts_FPGA)-1  CountFromType=Initial value  CountFrom=0  CountResetPort=off  CountLoadPort=off  CountEnbPort=off  CountDirPort=off  CountDataType=Unsigned  CountWordLen=32  CountFracLen=0  CountSampTime=Ts_FPGA
  pulses : Outport
  wires:
  PWM_counter/1 -> Compare To Constant4/1
  Mux/1 -> pulses/1
  Compare To Constant4/1 -> Mux/1, Mux/4, Logical Operator/1  "S1,4"
  Logical Operator/1 -> Mux/3, Mux/2  "S2,3"

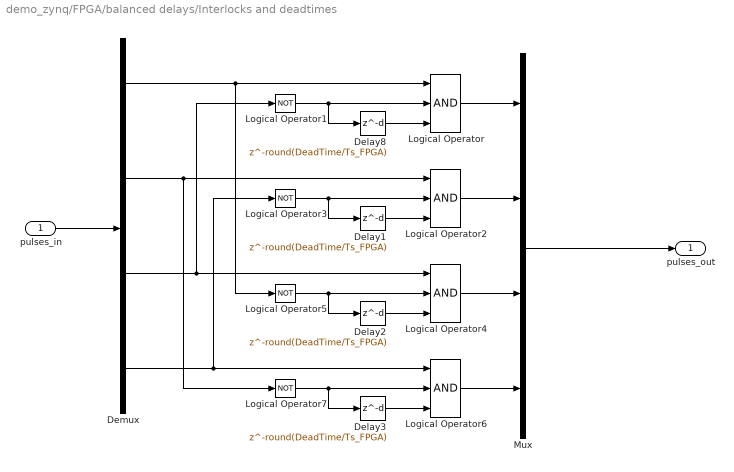
== system demo_zynq/FPGA/balanced delays/Interlocks and deadtimes ==
  pulses_in : Inport
  Delay{1..3,8} (4 alike) : Delay  DelayLength=round(DeadTime/Ts_FPGA)  InitialCondition=0
  Demux : Demux
  Logical Operator{,2,4,6} (4 alike) : Logic  Inputs=3  IconShape=distinctive  AllPortsSameDT=off  OutDataTypeStr=boolean
  Logical Operator{1,3,5,7} (4 alike) : Logic  Operator=NOT  IconShape=distinctive  AllPortsSameDT=off  OutDataTypeStr=boolean
  Mux : Mux
  pulses_out : Outport
  wires:
  pulses_in/1 -> Demux/1
  Demux/1 -> Logical Operator5/1, Logical Operator/1
  Demux/3 -> Logical Operator4/1, Logical Operator1/1
  Logical Operator1/1 -> Delay8/1, Logical Operator/2
  Delay8/1 -> Logical Operator/3
  Delay1/1 -> Logical Operator2/3
  Logical Operator3/1 -> Logical Operator2/2, Delay1/1
  Demux/2 -> Logical Operator7/1, Logical Operator2/1
  Delay2/1 -> Logical Operator4/3
  Logical Operator5/1 -> Logical Operator4/2, Delay2/1
  Logical Operator7/1 -> Delay3/1, Logical Operator6/2
  Delay3/1 -> Logical Operator6/3
  Demux/4 -> Logical Operator6/1, Logical Operator3/1
  Logical Operator/1 -> Mux/1
  Logical Operator2/1 -> Mux/2
  Logical Operator4/1 -> Mux/3
  Logical Operator6/1 -> Mux/4
  Mux/1 -> pulses_out/1

== system demo_zynq/FPGA/balanced delays/Ramp and sine generator ==
  note: Use only one implementation - comment out the other
  note: Sine calculation in fixed-point arithmetic
  note: Sine calculation in floating-point arithmetic
  clk : Inport
  Data Type Conversion : DataTypeConversion  Commented=on  OutDataTypeStr=single
  Data Type Conversion1 : DataTypeConversion  Commented=on  OutDataTypeStr=fixdt(1,32,30)
  Detect Increase : simulink/Logic and Bit Operations/Detect Increase  vinit=0.0  OutDataTypeStr=boolean
  Gain : Gain  Gain=1/round(0.02/Ts_ADC_sample) * (2*pi)
  HDL Counter : hdlsllib/Sources/HDL Counter  CountType=Free running  CountInit=0  CountStep=1  CountMax=25  CountFromType=Initial value  CountFrom=0  CountResetPort=off  CountLoadPort=off  CountEnbPort=on  CountDirPort=off  CountDataType=Unsigned  CountWordLen=10  CountFracLen=0  CountSampTime=Ts_FPGA
      settings: SourceProductName=Simulink
  HDL Counter1 : hdlsllib/Sources/HDL Counter  CountType=Count limited  CountInit=0  CountStep=1  CountMax=round(0.02/Ts_ADC_sample)-1  CountFromType=Initial value  CountFrom=0  CountResetPort=off  CountLoadPort=off  CountEnbPort=on  CountDirPort=off  CountDataType=Signed  CountWordLen=12  CountFracLen=0  CountSampTime=Ts_FPGA
      settings: SourceProductName=Simulink
  Sin : Trigonometry  Commented=on
  Sin Cordic : Trigonometry  ApproximationMethod=CORDIC
  Ramp : Outport
  Sine : Outport  Port=2
  wires:
  Detect Increase/1 -> HDL Counter1/1, HDL Counter/1
  HDL Counter/1 -> Ramp/1
  clk/1 -> Detect Increase/1
  HDL Counter1/1 -> Gain/1
  Gain/1 -> Sin Cordic/1, Data Type Conversion/1
  Data Type Conversion/1 -> Sin/1
  Sin/1 -> Data Type Conversion1/1
  Data Type Conversion1/1 -> ?
  Sin Cordic/1 -> Sine/1

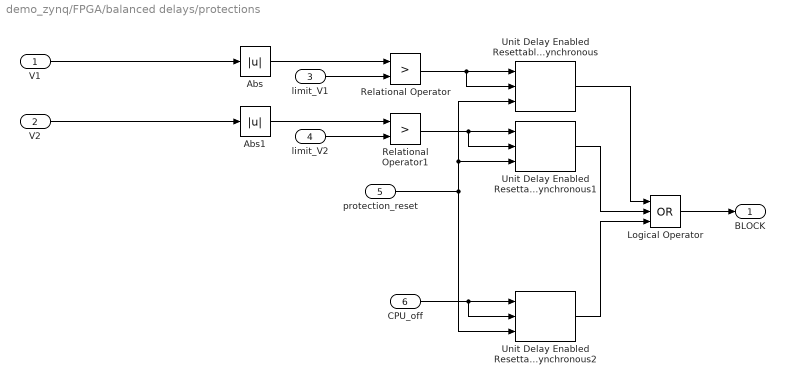
== system demo_zynq/FPGA/balanced delays/protections ==
  V1 : Inport
  V2 : Inport  Port=2
  limit_V1 : Inport  Port=3  OutDataTypeStr=fixdt(1,32,29)  SampleTime=Ts_FPGA
  limit_V2 : Inport  Port=4  OutDataTypeStr=fixdt(1,32,29)  SampleTime=Ts_FPGA
  protection_reset : Inport  Port=5  OutDataTypeStr=boolean  SampleTime=Ts_FPGA
  CPU_off : Inport  Port=6  OutDataTypeStr=boolean  SampleTime=Ts_FPGA
  Abs : Abs
  Abs1 : Abs
  Logical Operator : Logic  Operator=OR  Inputs=3  AllPortsSameDT=off  OutDataTypeStr=boolean
  Relational Operator : RelationalOperator  Operator=>  OutDataTypeStr=boolean  RndMeth=Nearest
  Relational Operator1 : RelationalOperator  Operator=>  OutDataTypeStr=boolean  RndMeth=Nearest
  Unit Delay Enabled Resettable Synchronous : hdlsllib/Discrete/Unit Delay Enabled Resettable Synchronous  InitialCondition=0.0  SampleTime=-1
      settings: SourceProductName=Simulink  SourceProductBaseCode=SL
  Unit Delay Enabled Resettable Synchronous1 : hdlsllib/Discrete/Unit Delay Enabled Resettable Synchronous  InitialCondition=0.0  SampleTime=-1
      settings: SourceProductName=Simulink  SourceProductBaseCode=SL
  Unit Delay Enabled Resettable Synchronous2 : hdlsllib/Discrete/Unit Delay Enabled Resettable Synchronous  InitialCondition=0.0  SampleTime=-1
      settings: SourceProductName=Simulink  SourceProductBaseCode=SL
  BLOCK : Outport
  wires:
  limit_V1/1 -> Relational Operator/2
  Abs/1 -> Relational Operator/1
  Unit Delay Enabled Resettable Synchronous/1 -> Logical Operator/1
  V2/1 -> Abs1/1
  Unit Delay Enabled Resettable Synchronous1/1 -> Logical Operator/2
  limit_V2/1 -> Relational Operator1/2
  Abs1/1 -> Relational Operator1/1
  Relational Operator/1 -> Unit Delay Enabled Resettable Synchronous/2, Unit Delay Enabled Resettable Synchronous/1
  Relational Operator1/1 -> Unit Delay Enabled Resettable Synchronous1/1, Unit Delay Enabled Resettable Synchronous1/2
  V1/1 -> Abs/1
  CPU_off/1 -> Unit Delay Enabled Resettable Synchronous2/1, Unit Delay Enabled Resettable Synchronous2/2
  Unit Delay Enabled Resettable Synchronous2/1 -> Logical Operator/3
  protection_reset/1 -> Unit Delay Enabled Resettable Synchronous2/3, Unit Delay Enabled Resettable Synchronous1/3, Unit Delay Enabled Resettable Synchronous/3
  Logical Operator/1 -> BLOCK/1

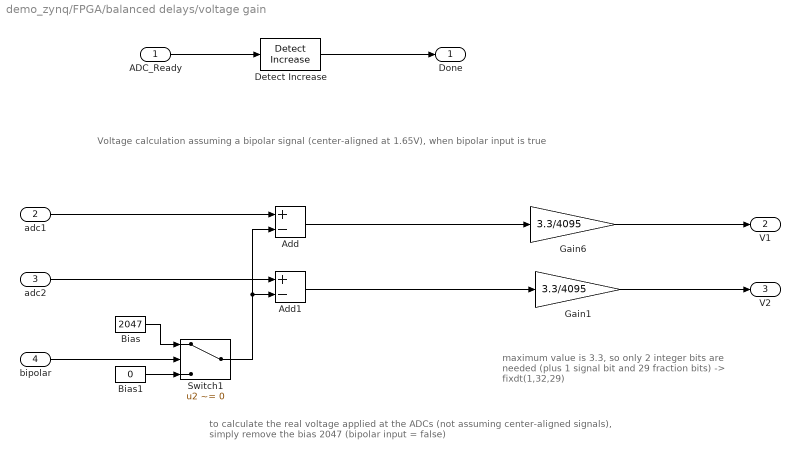
== system demo_zynq/FPGA/balanced delays/voltage gain ==
  note: Voltage calculation assuming a bipolar signal
      | (center-aligned at 1.65V), when bipolar input is true
  note: maximum value is 3.3, so only 2 integer bits
      | are needed (plus 1 signal bit and 29 fraction bits)
      | -> fixdt(1,32,29)
  note: to calculate the real voltage applied at the ADCs (not assuming center-aligned signals),
      | simply remove the bias 2047   (bipolar input = false)
  ADC_Ready : Inport
  adc1 : Inport  Port=2
  adc2 : Inport  Port=3
  bipolar : Inport  Port=4
  Add : Sum  Inputs=+-  AccumDataTypeStr=int32
  Add1 : Sum  Inputs=+-  AccumDataTypeStr=int32
  Bias : Constant  Value=2047  OutDataTypeStr=int32  SampleTime=-1
  Bias1 : Constant  Value=0  OutDataTypeStr=int32  SampleTime=-1
  Detect Increase : simulink/Logic and Bit Operations/Detect Increase  vinit=0.0  OutDataTypeStr=boolean
  Gain1 : Gain  Gain=3.3/4095  OutDataTypeStr=fixdt(1,32,29)
  Gain6 : Gain  Gain=3.3/4095  OutDataTypeStr=fixdt(1,32,29)  SaturateOnIntegerOverflow=on
  Switch1 : Switch  Criteria=u2 ~= 0
  "  Done" : Outport
  V1 : Outport  Port=2
  "  V2" : Outport  Port=3
  wires:
  ADC_Ready/1 -> Detect Increase/1
  Gain6/1 -> V1/1
  Gain1/1 -> "  V2"/1
  Add/1 -> Gain6/1
  Switch1/1 -> Add/2, Add1/2
  Detect Increase/1 -> "  Done"/1
  adc1/1 -> Add/1
  adc2/1 -> Add1/1
  Add1/1 -> Gain1/1
  Bias/1 -> Switch1/1
  bipolar/1 -> Switch1/2
  Bias1/1 -> Switch1/3

== system demo_zynq/FPGA/balanced delays/FIFO_DataAcquisition/Debug_FIFO ==
  DataIn : Inport
  enableFIFO : Inport  Port=2  OutDataTypeStr=boolean
  pushFIFO : Inport  Port=3  OutDataTypeStr=boolean
  enableRead : Inport  Port=4  OutDataTypeStr=boolean
  popFIFO : Inport  Port=5  OutDataTypeStr=boolean
  Constant : Constant  Value=0  OutDataTypeStr=Inherit: Inherit via back propagation  SampleTime=-1
  FIFO_Controller : MATLAB Function  TreatAsAtomicUnit=on
  HDL FIFO : hdlsllib/HDL RAMs/HDL FIFO  fifo_size=FIFO_length  mode=Classic  ratio=1  push_msg=Ignore  pop_msg=Ignore  show_empty=on  show_full=on  show_num=on  LabelModeActiveChoice_Mode=Classic
      settings: SourceProductName=Simulink  SourceProductBaseCode=SL
  Switch : Switch  Criteria=u2 > Threshold
  DataOut : Outport  VectorParamsAs1DForOutWhenUnconnected=off
  FifoNum : Outport  Port=2  VectorParamsAs1DForOutWhenUnconnected=off
  wires:
  HDL FIFO/2 -> FIFO_Controller/6(fifo_empty)
  HDL FIFO/3 -> FIFO_Controller/5(fifo_full)
  HDL FIFO/4 -> FifoNum/1  "num"
  FIFO_Controller/1(fifo_push) -> HDL FIFO/2
  HDL FIFO/1 -> Switch/3
  DataIn/1 -> HDL FIFO/1  "data_in"
  popFIFO/1 -> FIFO_Controller/4(popFIFO)
  FIFO_Controller/2(fifo_pop) -> HDL FIFO/3
  pushFIFO/1 -> FIFO_Controller/2(pushFIFO)
  enableFIFO/1 -> FIFO_Controller/1(enableFIFO)
  Switch/1 -> DataOut/1  "data_out"
  enableRead/1 -> FIFO_Controller/3(enableRead)  "enableIn"
  Constant/1 -> Switch/1
  FIFO_Controller/3(ignore) -> Switch/2

== system demo_zynq/FPGA/balanced delays/FIFO_DataAcquisition/Debug_FIFO1 ==
  DataIn : Inport
  enableFIFO : Inport  Port=2  OutDataTypeStr=boolean
  pushFIFO : Inport  Port=3  OutDataTypeStr=boolean
  enableRead : Inport  Port=4  OutDataTypeStr=boolean
  popFIFO : Inport  Port=5  OutDataTypeStr=boolean
  Constant : Constant  Value=0  OutDataTypeStr=Inherit: Inherit via back propagation  SampleTime=-1
  FIFO_Controller : MATLAB Function  TreatAsAtomicUnit=on
  HDL FIFO : hdlsllib/HDL RAMs/HDL FIFO  fifo_size=FIFO_length  mode=Classic  ratio=1  push_msg=Ignore  pop_msg=Ignore  show_empty=on  show_full=on  show_num=on  LabelModeActiveChoice_Mode=Classic
      settings: SourceProductName=Simulink  SourceProductBaseCode=SL
  Switch : Switch  Criteria=u2 > Threshold
  DataOut : Outport  VectorParamsAs1DForOutWhenUnconnected=off
  FifoNum : Outport  Port=2  VectorParamsAs1DForOutWhenUnconnected=off
  wires:
  FIFO_Controller/3(ignore) -> Switch/2
  Constant/1 -> Switch/1
  enableRead/1 -> FIFO_Controller/3(enableRead)  "enableIn"
  Switch/1 -> DataOut/1  "data_out"
  enableFIFO/1 -> FIFO_Controller/1(enableFIFO)
  pushFIFO/1 -> FIFO_Controller/2(pushFIFO)
  FIFO_Controller/2(fifo_pop) -> HDL FIFO/3
  popFIFO/1 -> FIFO_Controller/4(popFIFO)
  DataIn/1 -> HDL FIFO/1  "data_in"
  HDL FIFO/1 -> Switch/3
  FIFO_Controller/1(fifo_push) -> HDL FIFO/2
  HDL FIFO/4 -> FifoNum/1  "num"
  HDL FIFO/3 -> FIFO_Controller/5(fifo_full)
  HDL FIFO/2 -> FIFO_Controller/6(fifo_empty)

== system demo_zynq/FPGA/balanced delays/FIFO_DataAcquisition/Debug_FIFO2 ==
  DataIn : Inport
  enableFIFO : Inport  Port=2  OutDataTypeStr=boolean
  pushFIFO : Inport  Port=3  OutDataTypeStr=boolean
  enableRead : Inport  Port=4  OutDataTypeStr=boolean
  popFIFO : Inport  Port=5  OutDataTypeStr=boolean
  Constant : Constant  Value=0  OutDataTypeStr=Inherit: Inherit via back propagation  SampleTime=-1
  FIFO_Controller : MATLAB Function  TreatAsAtomicUnit=on
  HDL FIFO : hdlsllib/HDL RAMs/HDL FIFO  fifo_size=FIFO_length  mode=Classic  ratio=1  push_msg=Ignore  pop_msg=Ignore  show_empty=on  show_full=on  show_num=on  LabelModeActiveChoice_Mode=Classic
      settings: SourceProductName=Simulink  SourceProductBaseCode=SL
  Switch : Switch  Criteria=u2 > Threshold
  DataOut : Outport  VectorParamsAs1DForOutWhenUnconnected=off
  FifoNum : Outport  Port=2  VectorParamsAs1DForOutWhenUnconnected=off
  wires:
  HDL FIFO/2 -> FIFO_Controller/6(fifo_empty)
  HDL FIFO/3 -> FIFO_Controller/5(fifo_full)
  HDL FIFO/4 -> FifoNum/1  "num"
  FIFO_Controller/1(fifo_push) -> HDL FIFO/2
  HDL FIFO/1 -> Switch/3
  DataIn/1 -> HDL FIFO/1  "data_in"
  popFIFO/1 -> FIFO_Controller/4(popFIFO)
  FIFO_Controller/2(fifo_pop) -> HDL FIFO/3
  pushFIFO/1 -> FIFO_Controller/2(pushFIFO)
  enableFIFO/1 -> FIFO_Controller/1(enableFIFO)
  Switch/1 -> DataOut/1  "data_out"
  enableRead/1 -> FIFO_Controller/3(enableRead)  "enableIn"
  Constant/1 -> Switch/1
  FIFO_Controller/3(ignore) -> Switch/2

== system demo_zynq/FPGA/balanced delays/FIFO_DataAcquisition/Debug_FIFO3 ==
  DataIn : Inport
  enableFIFO : Inport  Port=2  OutDataTypeStr=boolean
  pushFIFO : Inport  Port=3  OutDataTypeStr=boolean
  enableRead : Inport  Port=4  OutDataTypeStr=boolean
  popFIFO : Inport  Port=5  OutDataTypeStr=boolean
  Constant : Constant  Value=0  OutDataTypeStr=Inherit: Inherit via back propagation  SampleTime=-1
  FIFO_Controller : MATLAB Function  TreatAsAtomicUnit=on
  HDL FIFO : hdlsllib/HDL RAMs/HDL FIFO  fifo_size=FIFO_length  mode=Classic  ratio=1  push_msg=Ignore  pop_msg=Ignore  show_empty=on  show_full=on  show_num=on  LabelModeActiveChoice_Mode=Classic
      settings: SourceProductName=Simulink  SourceProductBaseCode=SL
  Switch : Switch  Criteria=u2 > Threshold
  DataOut : Outport  VectorParamsAs1DForOutWhenUnconnected=off
  FifoNum : Outport  Port=2  VectorParamsAs1DForOutWhenUnconnected=off
  wires:
  FIFO_Controller/3(ignore) -> Switch/2
  Constant/1 -> Switch/1
  enableRead/1 -> FIFO_Controller/3(enableRead)  "enableIn"
  Switch/1 -> DataOut/1  "data_out"
  enableFIFO/1 -> FIFO_Controller/1(enableFIFO)
  pushFIFO/1 -> FIFO_Controller/2(pushFIFO)
  FIFO_Controller/2(fifo_pop) -> HDL FIFO/3
  popFIFO/1 -> FIFO_Controller/4(popFIFO)
  DataIn/1 -> HDL FIFO/1  "data_in"
  HDL FIFO/1 -> Switch/3
  FIFO_Controller/1(fifo_push) -> HDL FIFO/2
  HDL FIFO/4 -> FifoNum/1  "num"
  HDL FIFO/3 -> FIFO_Controller/5(fifo_full)
  HDL FIFO/2 -> FIFO_Controller/6(fifo_empty)

== system demo_zynq/FPGA/balanced delays/FIFO_DataAcquisition/delay start of window ==
  push : Inport
  enableIn : Inport  Port=2
  delay : Inport  Port=3
  Add : Sum  Inputs=+-  AccumDataTypeStr=int32  SaturateOnIntegerOverflow=on  OutDataTypeStr=Inherit: Same as first input
  Constant : Constant  Value=FIFO_length-1  OutDataTypeStr=uint32  SampleTime=Ts_FPGA
  HDL Counter : hdlsllib/Sources/HDL Counter  CountType=Free running  CountInit=0  CountStep=1  CountMax=25  CountFromType=Initial value  CountFrom=0  CountResetPort=on  CountLoadPort=off  CountEnbPort=on  CountDirPort=off  CountDataType=Unsigned  CountWordLen=32  CountFracLen=0  CountSampTime=1
      settings: SourceProductName=Simulink
  Logical Operator : Logic  Inputs=3  AllPortsSameDT=off  OutDataTypeStr=boolean
  Logical Operator1 : Logic  Operator=NOT  Inputs=3  AllPortsSameDT=off  OutDataTypeStr=boolean
  Logical Operator2 : Logic  Operator=NOT  Inputs=3  AllPortsSameDT=off  OutDataTypeStr=boolean
  Relational Operator : RelationalOperator  Operator=>  OutDataTypeStr=boolean  RndMeth=Simplest
  enable : Outport
  wires:
  Relational Operator/1 -> Logical Operator2/1, enable/1  "enable"
  HDL Counter/1 -> Relational Operator/1  "count"
  push/1 -> Logical Operator/1
  Logical Operator1/1 -> HDL Counter/1
  enableIn/1 -> Logical Operator/2, Logical Operator1/1
  Logical Operator/1 -> HDL Counter/2
  Constant/1 -> Add/1
  Add/1 -> Relational Operator/2
  delay/1 -> Add/2
  Logical Operator2/1 -> Logical Operator/3

== stateflow chart demo_zynq/FPGA/ADC/Chart ==
  settings: executeAtInitialization=1
  state WAIT
    data = 0;
    data1 = 0;
    EoC = false;
    EoA = false;
  state WAIT2
    ADC0 = data;
    ADC1 = data1;
    EoC = true;
  state ZEROS
    %if(D0)
    %    error = true;
    %end
    i=i+1;
  state READ_BITS
    %data = bitset(data, i, D0);
    EoA = true;
    data = bitsll(data,1);
    data = bitor(data, uint32(D0));
    data1 = bitsll(data1,1);
    data1 = bitor(data1, uint32(D1));
    i=i-1;
  (default) -> WAIT
  WAIT2 -> WAIT : [CS]
  WAIT -> ZEROS : [~CS]
      | {i=0}
  READ_BITS -> WAIT2 : [i==0]
  ZEROS -> READ_BITS : [i==3]
      | {i=12}
  data: EoC output boolean size=1 =false; CS input boolean size=1; ADC0 output uint32 size=1 =uint32(0); i local uint8 =uint8(0); data local uint32 =uint32(0); ADC1 output uint32 size=1 =uint32(0); data1 local uint32 size=1 =uint32(0); D0 input boolean size=1; D1 input boolean size=1; EoA output boolean =false
  events: Enable input RISING_EDGE_EVENT
